simulink model "MAIN_UAVSIM_Simulink"  (R2022a)
settings: Solver=FixedStepAuto  StartTime=0.0  StopTime=inf  RelTol=1e-3  EnableMultiTasking=on
undefined symbols (not defined in the file or in its folder): altREF, latREF, lonREF
libraries: slrealtimeutilitieslib x3, dspnetwork x2, slrealtimeiplib x1, aerolibanimutils x1, deeplib x1
settings Model: Creator=WiSE EFS  LastModifiedBy=Adi Kelvianto
settings SolverCC: AlgebraicLoopSolver=TrustRegion
settings DataIOCC: SaveFormat=Array  SignalLoggingSaveFormat=ModelDataLogs  SaveOutput=off  SaveTime=off  ReturnWorkspaceOutputs=off
settings OptimizationCC: ExpressionDepthLimit=2147483647  LifeSpan=inf
settings DebuggingCC: UnderspecifiedInitializationDetection=Classic  MergeDetectMultiDrivingBlocksExec=none  SolverPrmCheckMsg=warning  InheritedTsInSrcMsg=none  MultiTaskCondExecSysMsg=none  MultiTaskRateTransMsg=warning  SigSpecEnsureSampleTimeMsg=none  FcnCallInpInsideContextMsg=warning  UnconnectedInputMsg=warning  UnconnectedOutputMsg=warning  UnconnectedLineMsg=warning  StateNameClashWarn=warning  SFUnexpectedBacktrackingDiag=warning  SFNoUnconditionalDefaultTransitionDiag=warning  SFExecutionAtInitializationDiag=none  SFMachineParentedDataDiag=warning  ArithmeticOperatorsInVariantConditions=warning
settings HardwareCC: ProdBitPerPointer=32  ProdBitPerSizeT=32  ProdBitPerPtrDiffT=32  ProdLargestAtomicFloat=None  ProdIntDivRoundTo=Undefined  ProdEndianess=Unspecified  ProdWordSize=32  ProdHWDeviceType=32-bit Generic
settings ModelReferenceCC: PropagateSignalLabelsOutOfModel=off
settings SFSimCC: SimUseLocalCustomCode=off  SimParseCustomCode=off  CustomCodeUndefinedFunction=UseInterfaceOnly  SimTargetLang=C++
settings RTWCC: RTWUseLocalCustomCode=off  TargetLang=C++  DLArmComputeVersion=19.05
settings CodeAppCC: StateflowObjectComments=on
settings GRTTargetCC: TargetLangStandard=C89/C90 (ANSI)  CombineOutputUpdateFcns=off  GRTInterface=on
settings ConfigComp: CovMetricSettings=dw  CovSaveCumulativeToWorkspaceVar=on  CovSaveSingleToWorkspaceVar=on  CovExternalEMLEnable=off  CovSFcnEnable=off

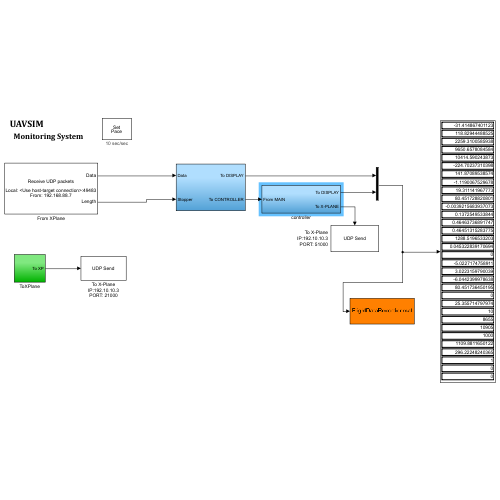
[thumbnail: Simulink's stored preview of the top-level diagram]
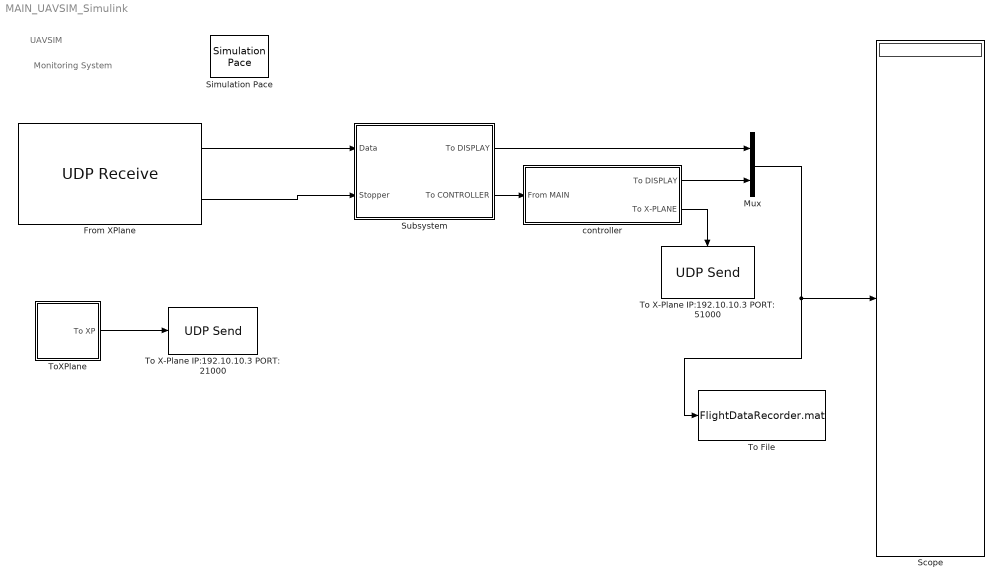
== system MAIN_UAVSIM_Simulink ==
  note: UAVSIM
  note: Monitoring System
  From XPlane : slrealtimeiplib/UDP Receive  useHostTargetConn=on  ipAddress=10.10.10.15  localPort=49483  rcvWidth=80  rcvFmAny=off  fmAddress=192.168.88.7  sampleTime=-1  enableMessage=off  maxPackets=1
      settings: SourceProductBaseCode=XP
  Mux : Mux  Inputs=2
  Scope : Display
  Simulation Pace : aerolibanimutils/Simulation Pace  SimulationPace=10  SleepMode=MATLAB Thread  OutputPaceError=off  SampleTime=-1
      settings: AttributesFormatString=%<SimulationPace> sec/sec
  Subsystem : Subsystem
  To File : ToFile  Filename=FlightDataRecorder.mat  MatrixName=FlightData  SampleTime=0.02
      settings: Decimation=50
  To X-Plane IP:192.10.10.3 PORT: 21000 : dspnetwork/UDP Send  remoteURL='192.168.88.7'  remotePort=49001  localURL='0.0.0.0'  localPortSource=Automatically determine  localPort=-1  sendBufferSize=8192  sampletime=-1  blockPlatform=[]  separateLengthPort=0
  To X-Plane IP:192.10.10.3 PORT: 51000 : dspnetwork/UDP Send  remoteURL='192.168.88.7'  remotePort=49000  localURL='0.0.0.0'  localPortSource=Automatically determine  localPort=-1  sendBufferSize=8192  sampletime=-1  blockPlatform=[]  separateLengthPort=0
  ToXPlane : Subsystem
  controller : Subsystem
  wires:
  From XPlane/1 -> Subsystem/1(Data)
  From XPlane/2 -> Subsystem/2(Stopper)
  ToXPlane/1(To XP) -> To X-Plane IP:192.10.10.3 PORT: 21000/1
  Subsystem/2(To CONTROLLER) -> controller/1(From MAIN)
  controller/2(To X-PLANE) -> To X-Plane IP:192.10.10.3 PORT: 51000/1
  Subsystem/1(To DISPLAY) -> Mux/1
  controller/1(To DISPLAY) -> Mux/2
  Mux/1 -> To File/1, Scope/1

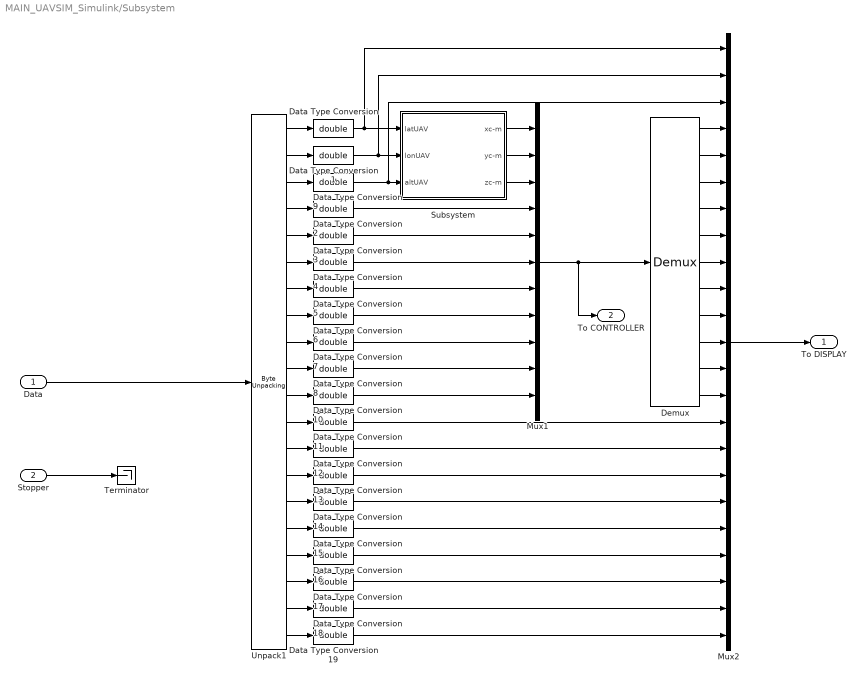
== system MAIN_UAVSIM_Simulink/Subsystem ==
  Data : Inport
  Stopper : Inport  Port=2
  Data Type Conversion{,1..19} (20 alike) : DataTypeConversion  OutDataTypeStr=double  SaturateOnIntegerOverflow=off  RndMeth=Floor
  Demux : Demux  Outputs=11
      settings: DisplayOption=none
  Mux1 : Mux  Inputs=11
  Mux2 : Mux  Inputs=23
  Subsystem : Subsystem
  Terminator : Terminator
  Unpack1 : slrealtimeutilitieslib/Byte Unpacking  MaskUnpackedDataTypes=dataType  MaskUnpackedDataSizes=dataChannel  MaskAlignment=4
      settings: SourceProductBaseCode=XP
  To DISPLAY : Outport
  To CONTROLLER : Outport  Port=2
  wires:
  Data/1 -> Unpack1/1
  Stopper/1 -> Terminator/1
  Unpack1/1 -> Data Type Conversion/1
  Unpack1/2 -> Data Type Conversion1/1
  Unpack1/3 -> Data Type Conversion9/1
  Unpack1/4 -> Data Type Conversion2/1
  Unpack1/5 -> Data Type Conversion3/1
  Unpack1/6 -> Data Type Conversion4/1
  Data Type Conversion1/1 -> Mux2/2, Subsystem/2(lonUAV)
  Data Type Conversion9/1 -> Mux2/3, Subsystem/3(altUAV)
  Subsystem/1(xc-m) -> Mux1/1
  Subsystem/2(yc-m) -> Mux1/2
  Subsystem/3(zc-m) -> Mux1/3
  Data Type Conversion2/1 -> Mux1/4
  Data Type Conversion3/1 -> Mux1/5
  Data Type Conversion4/1 -> Mux1/6
  Unpack1/7 -> Data Type Conversion5/1
  Unpack1/8 -> Data Type Conversion6/1
  Data Type Conversion6/1 -> Mux1/8
  Unpack1/9 -> Data Type Conversion7/1
  Data Type Conversion7/1 -> Mux1/9
  Unpack1/10 -> Data Type Conversion8/1
  Data Type Conversion8/1 -> Mux1/10
  Unpack1/11 -> Data Type Conversion10/1
  Data Type Conversion10/1 -> Mux1/11
  Unpack1/12 -> Data Type Conversion11/1
  Unpack1/13 -> Data Type Conversion12/1
  Unpack1/14 -> Data Type Conversion13/1
  Unpack1/15 -> Data Type Conversion14/1
  Unpack1/16 -> Data Type Conversion15/1
  Unpack1/17 -> Data Type Conversion16/1
  Unpack1/18 -> Data Type Conversion17/1
  Unpack1/19 -> Data Type Conversion18/1
  Unpack1/20 -> Data Type Conversion19/1
  Mux2/1 -> To DISPLAY/1
  Data Type Conversion5/1 -> Mux1/7
  Data Type Conversion/1 -> Mux2/1, Subsystem/1(latUAV)
  Data Type Conversion19/1 -> Mux2/23
  Data Type Conversion18/1 -> Mux2/22
  Data Type Conversion17/1 -> Mux2/21
  Data Type Conversion16/1 -> Mux2/20
  Data Type Conversion15/1 -> Mux2/19
  Data Type Conversion14/1 -> Mux2/18
  Data Type Conversion13/1 -> Mux2/17
  Data Type Conversion12/1 -> Mux2/16
  Data Type Conversion11/1 -> Mux2/15
  Mux1/1 -> To CONTROLLER/1, Demux/1
  Demux/11 -> Mux2/14
  Demux/10 -> Mux2/13
  Demux/9 -> Mux2/12
  Demux/8 -> Mux2/11
  Demux/7 -> Mux2/10
  Demux/6 -> Mux2/9
  Demux/5 -> Mux2/8
  Demux/4 -> Mux2/7
  Demux/3 -> Mux2/6
  Demux/2 -> Mux2/5
  Demux/1 -> Mux2/4

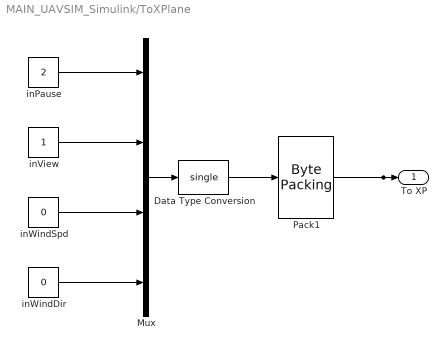
== system MAIN_UAVSIM_Simulink/ToXPlane ==
  Data Type Conversion : DataTypeConversion  OutDataTypeStr=single  SaturateOnIntegerOverflow=off  RndMeth=Floor
  Mux : Mux
  Pack1 : slrealtimeutilitieslib/Byte Packing  MaskPackedDataType=uint8  MaskUnpackedDataTypes={'single'}  MaskAlignment=4
  inPause : Constant  Value=2  SampleTime=0
  inView : Constant  SampleTime=0
  inWindDir : Constant  Value=0  SampleTime=0
  inWindSpd : Constant  Value=0  SampleTime=0
  To XP : Outport
  wires:
  Mux/1 -> Data Type Conversion/1
  Pack1/1 -> To XP/1
  inPause/1 -> Mux/1
  inView/1 -> Mux/2
  inWindSpd/1 -> Mux/3
  inWindDir/1 -> Mux/4
  Data Type Conversion/1 -> Pack1/1

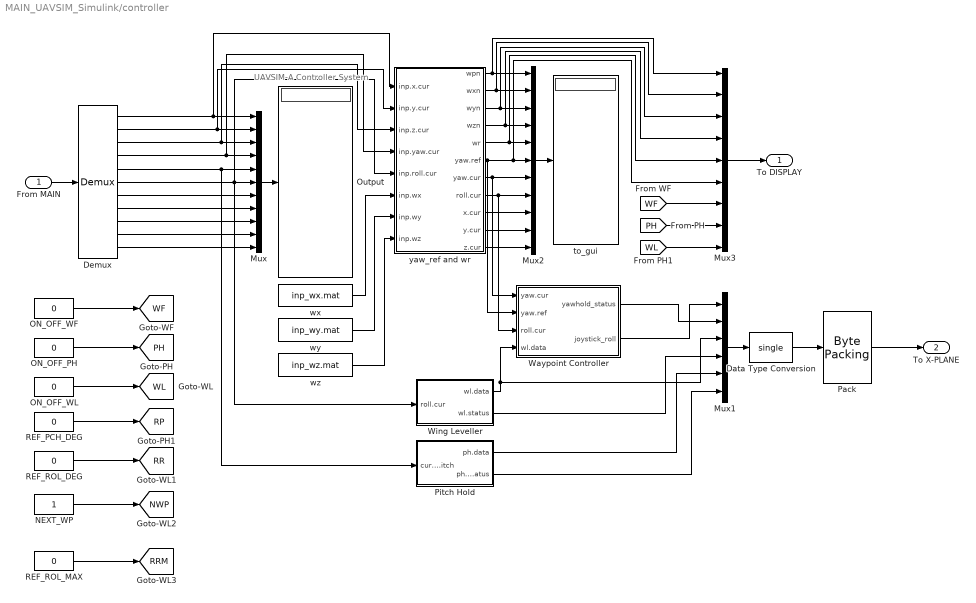
== system MAIN_UAVSIM_Simulink/controller ==
  note: UAVSIM-A
      | Controller System
  From MAIN : Inport
  Data Type Conversion : DataTypeConversion  OutDataTypeStr=single  SaturateOnIntegerOverflow=off  RndMeth=Floor
  Demux : Demux  Outputs=11
      settings: DisplayOption=none
  Mux : Mux  Inputs=11
  Mux1 : Mux  Inputs=6
  Mux2 : Mux  Inputs=11
  Mux3 : Mux  Inputs=9
  NEXT_WP : Constant  SampleTime=0
  ON_OFF_PH : Constant  Value=0  SampleTime=0
  ON_OFF_WF : Constant  Value=0  SampleTime=0
  ON_OFF_WL : Constant  Value=0  SampleTime=0
  Output : Display
  Pack : slrealtimeutilitieslib/Byte Packing  MaskPackedDataType=uint8  MaskUnpackedDataTypes={'single'}  MaskAlignment=4
  Pitch Hold : Subsystem
  REF_PCH_DEG : Constant  Value=0  SampleTime=0
  REF_ROL_DEG : Constant  Value=0  SampleTime=0
  REF_ROL_MAX : Constant  Value=0  SampleTime=0
  Waypoint Controller : Subsystem
  Wing Leveller : Subsystem
  to_gui : Display
  wx : FromFile  FileName=inp_wx.mat  SampleTime=0  ExtrapolationBeforeFirstDataPoint=Hold first value  ExtrapolationAfterLastDataPoint=Hold last value
  wy : FromFile  FileName=inp_wy.mat  SampleTime=0  ExtrapolationBeforeFirstDataPoint=Hold first value  ExtrapolationAfterLastDataPoint=Hold last value
  wz : FromFile  FileName=inp_wz.mat  SampleTime=0  ExtrapolationBeforeFirstDataPoint=Hold first value  ExtrapolationAfterLastDataPoint=Hold last value
  yaw_ref and wr : Subsystem
  To DISPLAY : Outport
  To X-PLANE : Outport  Port=2
  tag scope: NWP=global, PH=global, RP=global, RR=global, RRM=global, WF=global, WL=global
  wires:
  yaw_ref and wr/10(y.cur) -> Mux2/10
  yaw_ref and wr/9(x.cur) -> Mux2/9
  Waypoint Controller/1(yawhold_status) -> Mux1/2
  yaw_ref and wr/7(yaw.cur) -> Waypoint Controller/1(yaw.cur), Mux2/7
  Wing Leveller/2(wl.status) -> Mux1/4
  Wing Leveller/1(wl.data) -> Waypoint Controller/4(wl.data), Mux1/3
  ON_OFF_WL/1 -> [WL]
  ON_OFF_WF/1 -> [WF]
  yaw_ref and wr/5(wr) -> Mux2/5, Mux3/5
  yaw_ref and wr/2(wxn) -> Mux2/2, Mux3/2
  Mux/1 -> Output/1
  Demux/11 -> Mux/11
  Mux1/1 -> Data Type Conversion/1
  REF_PCH_DEG/1 -> [RP]
  Demux/1 -> Mux/1, yaw_ref and wr/1(inp.x.cur)
  yaw_ref and wr/11(z.cur) -> Mux2/11
  wz/1 -> yaw_ref and wr/8(inp.wz)
  NEXT_WP/1 -> [NWP]
  Demux/7 -> Mux/7
  yaw_ref and wr/8(roll.cur) -> Waypoint Controller/3(roll.cur), Mux2/8
  yaw_ref and wr/4(wzn) -> Mux2/4, Mux3/4
  Demux/2 -> Mux/2, yaw_ref and wr/2(inp.y.cur)
  [WL] -> Mux3/9
  Pitch Hold/2(ph.status) -> Mux1/6
  Mux2/1 -> to_gui/1
  Demux/5 -> Mux/5, Pitch Hold/1(cur.pitch)
  Demux/8 -> Mux/8
  REF_ROL_DEG/1 -> [RR]
  wx/1 -> yaw_ref and wr/6(inp.wx)
  Demux/4 -> Mux/4, yaw_ref and wr/4(inp.yaw.cur)
  Waypoint Controller/2(joystick_roll) -> Mux1/1
  yaw_ref and wr/6(yaw.ref) -> Waypoint Controller/2(yaw.ref), Mux2/6, Mux3/6
  Demux/3 -> Mux/3, yaw_ref and wr/3(inp.z.cur)
  Pitch Hold/1(ph.data) -> Mux1/5
  Demux/6 -> Mux/6, Wing Leveller/1(roll.cur), yaw_ref and wr/5(inp.roll.cur)
  wy/1 -> yaw_ref and wr/7(inp.wy)
  Data Type Conversion/1 -> Pack/1
  ON_OFF_PH/1 -> [PH]
  yaw_ref and wr/1(wpn) -> Mux2/1, Mux3/1
  Demux/9 -> Mux/9
  Demux/10 -> Mux/10
  [WF] -> Mux3/7
  [PH] -> Mux3/8
  yaw_ref and wr/3(wyn) -> Mux2/3, Mux3/3
  From MAIN/1 -> Demux/1
  Mux3/1 -> To DISPLAY/1
  Pack/1 -> To X-PLANE/1
  REF_ROL_MAX/1 -> [RRM]

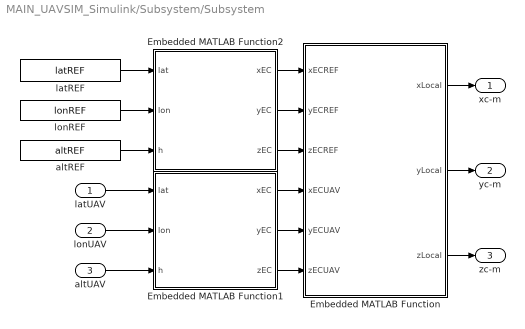
== system MAIN_UAVSIM_Simulink/Subsystem/Subsystem ==
  latUAV : Inport
  lonUAV : Inport  Port=2
  altUAV : Inport  Port=3
  Embedded MATLAB Function : MATLAB Function  TreatAsAtomicUnit=on
  Embedded MATLAB Function1 : MATLAB Function  TreatAsAtomicUnit=on
  Embedded MATLAB Function2 : MATLAB Function  TreatAsAtomicUnit=on
  altREF : Constant  Value=altREF  SampleTime=0.02
  latREF : Constant  Value=latREF  SampleTime=0.02
  lonREF : Constant  Value=lonREF  SampleTime=0.02
  xc-m : Outport
  yc-m : Outport  Port=2
  zc-m : Outport  Port=3
  wires:
  Embedded MATLAB Function/1(xLocal) -> xc-m/1
  Embedded MATLAB Function/3(zLocal) -> zc-m/1
  Embedded MATLAB Function/2(yLocal) -> yc-m/1
  latREF/1 -> Embedded MATLAB Function2/1(lat)
  lonREF/1 -> Embedded MATLAB Function2/2(lon)
  altREF/1 -> Embedded MATLAB Function2/3(h)
  Embedded MATLAB Function2/1(xEC) -> Embedded MATLAB Function/1(xECREF)
  Embedded MATLAB Function2/2(yEC) -> Embedded MATLAB Function/2(yECREF)
  Embedded MATLAB Function2/3(zEC) -> Embedded MATLAB Function/3(zECREF)
  Embedded MATLAB Function1/1(xEC) -> Embedded MATLAB Function/4(xECUAV)
  Embedded MATLAB Function1/2(yEC) -> Embedded MATLAB Function/5(yECUAV)
  Embedded MATLAB Function1/3(zEC) -> Embedded MATLAB Function/6(zECUAV)
  latUAV/1 -> Embedded MATLAB Function1/1(lat)
  lonUAV/1 -> Embedded MATLAB Function1/2(lon)
  altUAV/1 -> Embedded MATLAB Function1/3(h)

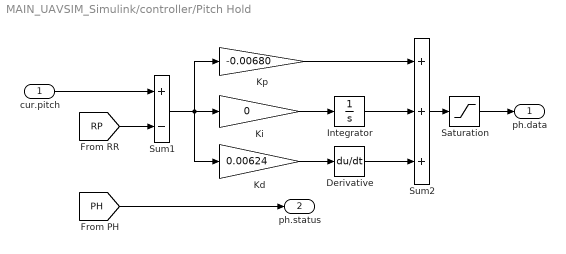
== system MAIN_UAVSIM_Simulink/controller/Pitch Hold ==
  cur.pitch : Inport
  Derivative : Derivative
  Integrator : Integrator
  Kd : Gain  Gain=0.00624
  Ki : Gain  Gain=0
  Kp : Gain  Gain=-0.00680
  Saturation : Saturate  UpperLimit=1  LowerLimit=-1
  Sum1 : Sum  Inputs=+-
  Sum2 : Sum  Inputs=+++
  ph.data : Outport
  ph.status : Outport  Port=2
  wires:
  Integrator/1 -> Sum2/2
  Ki/1 -> Integrator/1
  Kp/1 -> Sum2/1
  Sum2/1 -> Saturation/1
  Kd/1 -> Derivative/1
  Derivative/1 -> Sum2/3
  [PH] -> ph.status/1
  Sum1/1 -> Ki/1, Kp/1, Kd/1
  cur.pitch/1 -> Sum1/1
  Saturation/1 -> ph.data/1
  [RP] -> Sum1/2

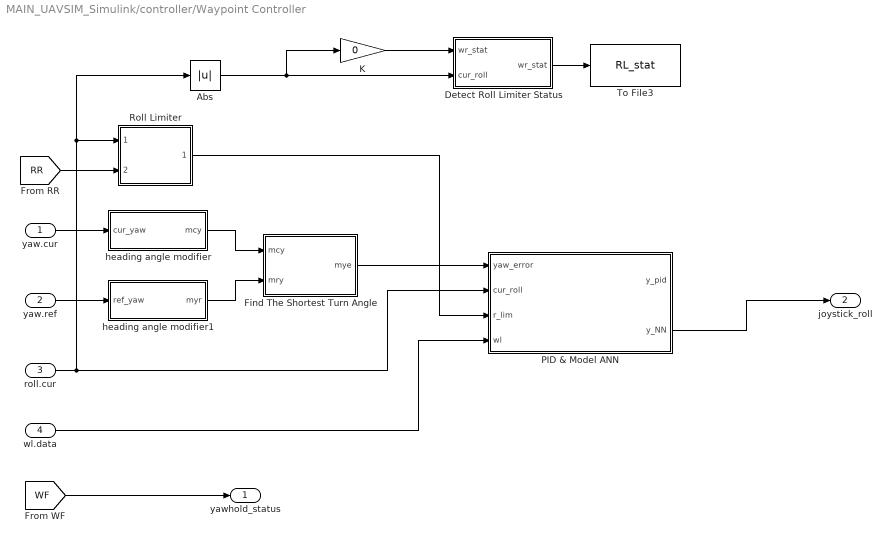
== system MAIN_UAVSIM_Simulink/controller/Waypoint Controller ==
  yaw.cur : Inport
  yaw.ref : Inport  Port=2
  roll.cur : Inport  Port=3
  wl.data : Inport  Port=4
  Abs : Abs  SaturateOnIntegerOverflow=off
  Detect Roll Limiter Status : MATLAB Function  TreatAsAtomicUnit=on
  Find The Shortest Turn Angle : MATLAB Function  TreatAsAtomicUnit=on
  K : Gain  Gain=0
  PID & Model ANN : Subsystem
  Roll Limiter : Subsystem
  To File3 : ToFile  Filename=RL_stat  MatrixName=RL_stat  SampleTime=0.02
      settings: Decimation=50
  heading angle modifier : MATLAB Function  TreatAsAtomicUnit=on
  heading angle modifier1 : MATLAB Function  TreatAsAtomicUnit=on
  yawhold_status : Outport
  joystick_roll : Outport  Port=2
  wires:
  [WF] -> yawhold_status/1
  [RR] -> Roll Limiter/2(roll.ref.max)
  yaw.cur/1 -> heading angle modifier/1(cur_yaw)
  yaw.ref/1 -> heading angle modifier1/1(ref_yaw)
  K/1 -> Detect Roll Limiter Status/1("wr_stat ")
  roll.cur/1 -> Abs/1, Roll Limiter/1(roll.cur), PID & Model ANN/2(cur_roll)
  Abs/1 -> K/1, Detect Roll Limiter Status/2(cur_roll)
  Detect Roll Limiter Status/1(wr_stat) -> To File3/1
  wl.data/1 -> PID & Model ANN/4(wl)
  Roll Limiter/1(roll.lim) -> PID & Model ANN/3(r_lim)
  heading angle modifier/1(mcy) -> Find The Shortest Turn Angle/1(mcy)
  heading angle modifier1/1(myr) -> Find The Shortest Turn Angle/2(mry)
  Find The Shortest Turn Angle/1(mye) -> PID & Model ANN/1(yaw_error)
  PID & Model ANN/2(y_NN) -> joystick_roll/1

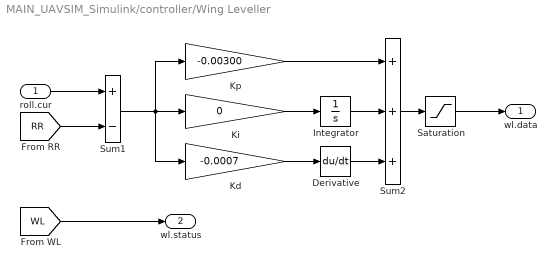
== system MAIN_UAVSIM_Simulink/controller/Wing Leveller ==
  roll.cur : Inport
  Derivative : Derivative
  Integrator : Integrator
  Kd : Gain  Gain=-0.0007
  Ki : Gain  Gain=0
  Kp : Gain  Gain=-0.00300
  Saturation : Saturate  UpperLimit=1  LowerLimit=-1
  Sum1 : Sum  Inputs=+-
  Sum2 : Sum  Inputs=+++
  wl.data : Outport
  wl.status : Outport  Port=2
  wires:
  Integrator/1 -> Sum2/2
  Ki/1 -> Integrator/1
  Kp/1 -> Sum2/1
  Sum2/1 -> Saturation/1
  Kd/1 -> Derivative/1
  Derivative/1 -> Sum2/3
  Sum1/1 -> Ki/1, Kp/1, Kd/1
  [RR] -> Sum1/2
  roll.cur/1 -> Sum1/1
  Saturation/1 -> wl.data/1
  [WL] -> wl.status/1

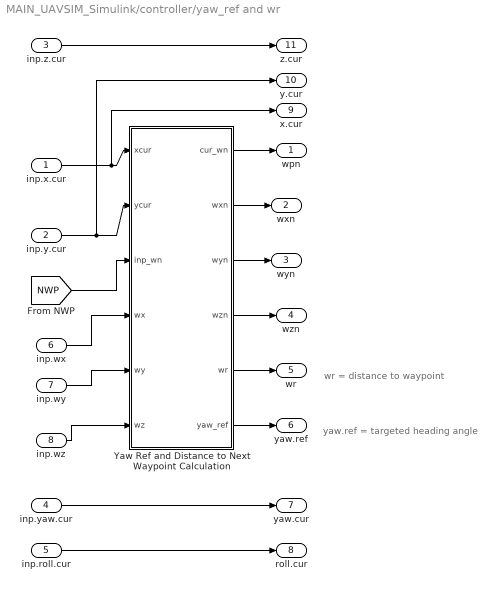
== system MAIN_UAVSIM_Simulink/controller/yaw_ref and wr ==
  note: yaw.ref = targeted heading angle
  note: wr = distance to waypoint
  inp.x.cur : Inport
  inp.y.cur : Inport  Port=2
  inp.z.cur : Inport  Port=3
  inp.yaw.cur : Inport  Port=4
  inp.roll.cur : Inport  Port=5
  inp.wx : Inport  Port=6
  inp.wy : Inport  Port=7
  inp.wz : Inport  Port=8
  Yaw Ref and Distance to Next Waypoint Calculation : MATLAB Function  TreatAsAtomicUnit=on
  wpn : Outport
  wxn : Outport  Port=2
  wyn : Outport  Port=3
  wzn : Outport  Port=4
  wr : Outport  Port=5
  yaw.ref : Outport  Port=6
  yaw.cur : Outport  Port=7
  roll.cur : Outport  Port=8
  x.cur : Outport  Port=9
  y.cur : Outport  Port=10
  z.cur : Outport  Port=11
  wires:
  inp.y.cur/1 -> Yaw Ref and Distance to Next Waypoint Calculation/2(ycur), y.cur/1
  inp.x.cur/1 -> Yaw Ref and Distance to Next Waypoint Calculation/1(xcur), x.cur/1
  [NWP] -> Yaw Ref and Distance to Next Waypoint Calculation/3(inp_wn)
  inp.yaw.cur/1 -> yaw.cur/1
  Yaw Ref and Distance to Next Waypoint Calculation/6(yaw_ref) -> yaw.ref/1
  inp.roll.cur/1 -> roll.cur/1
  Yaw Ref and Distance to Next Waypoint Calculation/1(cur_wn) -> wpn/1
  Yaw Ref and Distance to Next Waypoint Calculation/2(wxn) -> wxn/1
  Yaw Ref and Distance to Next Waypoint Calculation/3(wyn) -> wyn/1
  Yaw Ref and Distance to Next Waypoint Calculation/4(wzn) -> wzn/1
  Yaw Ref and Distance to Next Waypoint Calculation/5(wr) -> wr/1
  inp.z.cur/1 -> z.cur/1
  inp.wx/1 -> Yaw Ref and Distance to Next Waypoint Calculation/4(wx)
  inp.wy/1 -> Yaw Ref and Distance to Next Waypoint Calculation/5(wy)
  inp.wz/1 -> Yaw Ref and Distance to Next Waypoint Calculation/6(wz)

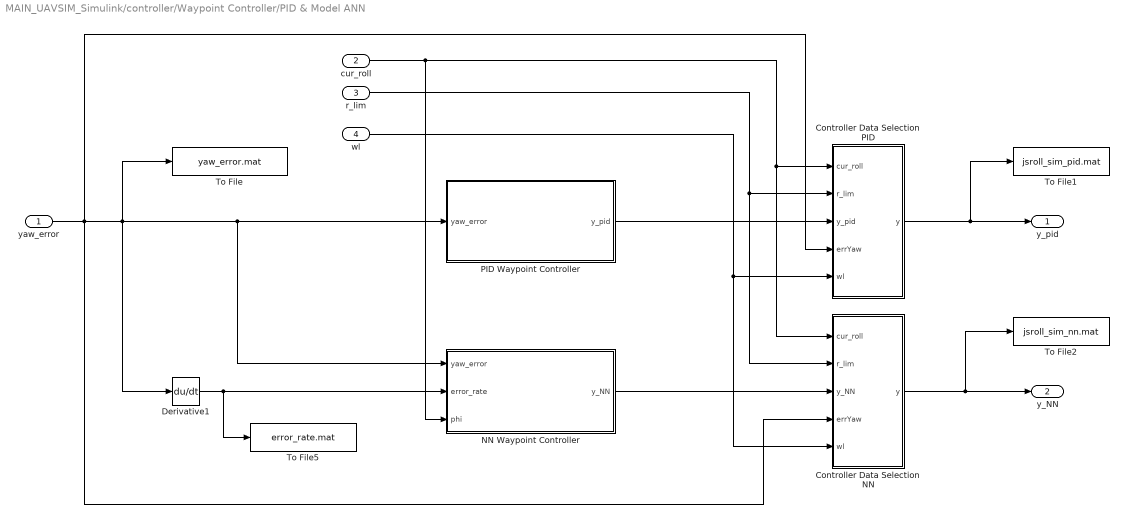
== system MAIN_UAVSIM_Simulink/controller/Waypoint Controller/PID & Model ANN ==
  yaw_error : Inport
  cur_roll : Inport  Port=2
  r_lim : Inport  Port=3
  wl : Inport  Port=4
  Controller Data Selection NN : MATLAB Function  TreatAsAtomicUnit=on
  Controller Data Selection PID : MATLAB Function  TreatAsAtomicUnit=on
  Derivative1 : Derivative
  NN Waypoint Controller : Subsystem
  PID Waypoint Controller : Subsystem
  To File : ToFile  Filename=yaw_error.mat  MatrixName=yaw_error  SampleTime=0.02
      settings: Decimation=50
  To File1 : ToFile  Filename=jsroll_sim_pid.mat  MatrixName=jsroll_sim_pid  SampleTime=0.02
      settings: Decimation=50
  To File2 : ToFile  Filename=jsroll_sim_nn.mat  MatrixName=jsroll_sim_nn  SampleTime=0.02
      settings: Decimation=50
  To File5 : ToFile  Filename=error_rate.mat  MatrixName=error_rate  SampleTime=0.02
      settings: Decimation=50
  y_pid : Outport
  y_NN : Outport  Port=2
  wires:
  PID Waypoint Controller/1(y_pid) -> Controller Data Selection PID/3(y_pid)
  cur_roll/1 -> Controller Data Selection NN/1(cur_roll), Controller Data Selection PID/1(cur_roll), NN Waypoint Controller/3(phi)
  r_lim/1 -> Controller Data Selection NN/2(r_lim), Controller Data Selection PID/2(r_lim)
  wl/1 -> Controller Data Selection NN/5(wl), Controller Data Selection PID/5(wl)
  NN Waypoint Controller/1(y_NN) -> Controller Data Selection NN/3(y_NN)
  Controller Data Selection PID/1(y) -> To File1/1, y_pid/1
  Controller Data Selection NN/1(y) -> To File2/1, y_NN/1
  yaw_error/1 -> Controller Data Selection NN/4(errYaw), Controller Data Selection PID/4(errYaw), To File/1, Derivative1/1, NN Waypoint Controller/1(yaw_error), PID Waypoint Controller/1(yaw_error)
  Derivative1/1 -> To File5/1, NN Waypoint Controller/2(error_rate)

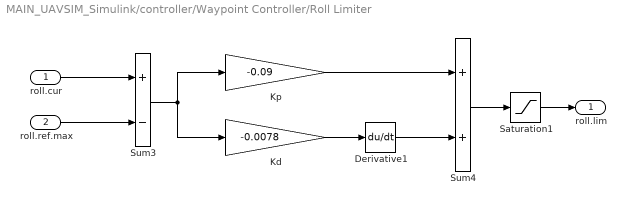
== system MAIN_UAVSIM_Simulink/controller/Waypoint Controller/Roll Limiter ==
  roll.cur : Inport
  roll.ref.max : Inport  Port=2
  Derivative1 : Derivative
  Kd : Gain  Gain=-0.0078
  Kp : Gain  Gain=-0.09
  Saturation1 : Saturate  UpperLimit=1  LowerLimit=-1
  Sum3 : Sum  Inputs=+-
  Sum4 : Sum
  roll.lim : Outport
  wires:
  Sum3/1 -> Kp/1, Kd/1
  Sum4/1 -> Saturation1/1
  Saturation1/1 -> roll.lim/1
  Derivative1/1 -> Sum4/2
  roll.ref.max/1 -> Sum3/2
  Kp/1 -> Sum4/1
  Kd/1 -> Derivative1/1
  roll.cur/1 -> Sum3/1

== system MAIN_UAVSIM_Simulink/controller/Waypoint Controller/PID & Model ANN/NN Waypoint Controller ==
  yaw_error : Inport
  error_rate : Inport  Port=2
  phi : Inport  Port=3
  Predict : deeplib/Predict  Network=Network from MAT-file  NetworkFunction=squeezenet  NetworkFilePath=D:\uavms\model_7aug_set4.mat  MiniBatchSize=1  InputDataFormats={ '', '' }  Predictions=on  Activations={}  ForceInterpretedSim=off  EnableDLNetwork=on
      settings: SourceProductBaseCode=NN
  Prepare Features : MATLAB Function  TreatAsAtomicUnit=on
  Saturation1 : Saturate  UpperLimit=1  LowerLimit=-1
  y_NN : Outport
  wires:
  error_rate/1 -> Prepare Features/1(error_rate)
  yaw_error/1 -> Prepare Features/2(yaw_error)
  phi/1 -> Prepare Features/3(phi)
  Prepare Features/1(features) -> Predict/1
  Saturation1/1 -> y_NN/1
  Predict/1 -> Saturation1/1

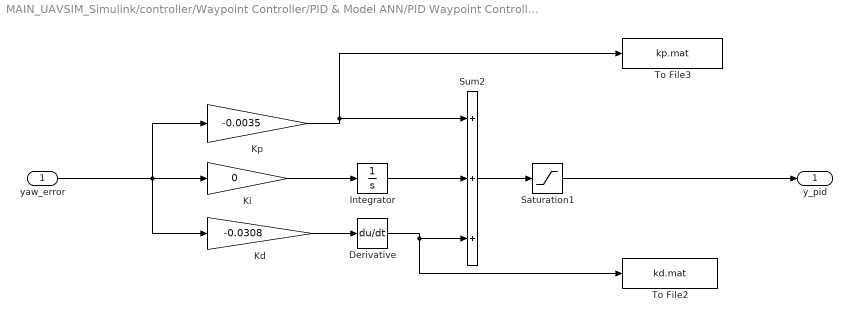
== system MAIN_UAVSIM_Simulink/controller/Waypoint Controller/PID & Model ANN/PID Waypoint Controller ==
  yaw_error : Inport
  Derivative : Derivative
  Integrator : Integrator
  Kd : Gain  Gain=-0.0308
  Ki : Gain  Gain=0
  Kp : Gain  Gain=-0.0035
  Saturation1 : Saturate  UpperLimit=1  LowerLimit=-1
  Sum2 : Sum  Inputs=+++
  To File2 : ToFile  Filename=kd.mat  MatrixName=kd  SampleTime=0.02
      settings: Decimation=50
  To File3 : ToFile  Filename=kp.mat  MatrixName=kp  SampleTime=0.02
      settings: Decimation=50
  y_pid : Outport
  wires:
  Sum2/1 -> Saturation1/1
  Derivative/1 -> Sum2/3, To File2/1
  Kp/1 -> To File3/1, Sum2/1
  Saturation1/1 -> y_pid/1
  Kd/1 -> Derivative/1
  yaw_error/1 -> Kd/1, Ki/1, Kp/1
  Ki/1 -> Integrator/1
  Integrator/1 -> Sum2/2

== matlab function MAIN_UAVSIM_Simulink/controller/yaw_ref and wr/Yaw Ref and Distance to Next Waypoint Calculation ==
  data: cur_wn output; wxn output; wyn output; wzn output; wr output; xcur input; yaw_ref output; ycur input; inp_wn input; wx input; wy input; wz input
function [cur_wn,wxn,wyn,wzn,wr,yaw_ref]  = fcn(xcur,ycur,inp_wn,wx,wy,wz)
%#eml

% Rectangular Waypoint
% wx = [3000;3000;8000;8000;3000;3000]; % The last data is for terminating only
% wy = [2000;8000;8000;2000;2000;2000]; % The last data is for terminating only
% wz = [500;600;500;500;500;700];

% Rectangular + X Waypoint
% wx = [3000;8000;3000;8000;3000;3000]; % The last data is for terminating only
% wy = [2000;2000;8000;8000;2000;2000]; % The last data is for terminating only
% wz = [500;600;500;500;500;700];

% Next waypoint coordinate
wxn = wx(inp_wn);
wyn = wy(inp_wn);
wzn = wz(inp_wn);

dx  = wx(inp_wn)-xcur;
dy  = wy(inp_wn)-ycur;

% Next waypoint heading angle and distance
yaw = 180*(atan2(dy,dx))/pi;
wr  = sqrt(dx^2 + dy^2);
    
if (dx < 0 && dy > 0)
    yaw_ref = 360 + (90-yaw);
else
    yaw_ref = 90-yaw;
end
   
cur_wn = inp_wn;

== matlab function MAIN_UAVSIM_Simulink/controller/Waypoint Controller/PID & Model ANN/NN Waypoint Controller/Prepare Features ==
  data: error_rate input; yaw_error input; features output; phi input
function features = fcn(error_rate, yaw_error, phi)
%#eml

features_raw = [error_rate, yaw_error,phi];
% Min Max value from train dataset for each features with sequnce of
% [error_rate, yaw_error, phi]

% set 1
%min_train = [-2.101, -17.924, -8.977];
%max_train = [1.543, 17.016, 9.541];

% set 2
%min_train = [-2.331, -93.562, -8.977];
%max_train = [5.371, 17.016, 32.265];

% set 3
%min_train = [-6.707, -17.924, -32.134];
%max_train = [4.487, 71.031, 9.541];

% set 4
min_train = [-6.707, -93.562, -32.134] ;
max_train = [5.559, 71.031, 34.303] ;

normalized = zeros(1,length(features_raw));

for i = 1:length(features_raw)
    normalized(i) = (features_raw(i)-min_train(i))/(max_train(i)-min_train(i));
end

features = normalized;
end

== matlab function MAIN_UAVSIM_Simulink/controller/Waypoint Controller/PID & Model ANN/Controller Data Selection NN ==
  data: cur_roll input; r_lim input; y output; y_NN input; errYaw input; wl input
function y = fcn(cur_roll,r_lim,y_NN,errYaw,wl)
%#eml
%diff

if abs(cur_roll)>=30
    y = r_lim;
else
    y = double(y_NN);
end
end

== matlab function MAIN_UAVSIM_Simulink/Subsystem/Subsystem/Embedded MATLAB Function1 ==
  data: lat input; lon input; xEC output; h input; yEC output; zEC output
function [xEC,yEC,zEC] = WGS2ECEF(lat,lon,h)

% Convert lat, long, height in WGS84 to ECEF X,Y,Z
% lat and long given in decimal degrees.
% altitude should be given in meters
a  = 6378137.0;       % earth semimajor axis in meters
f  = 1/298.257223563; % reciprocal flattening
e2 = 2*f -f^2;        % eccentricity squared
 
chi = sqrt(1-e2*(sind(lat)).^2);
xEC = (a./chi + h).*cosd(lat).*cosd(lon);
yEC = (a./chi + h).*cosd(lat).*sind(lon);
zEC = (a*(1-e2)./chi + h).*sind(lat);

== matlab function MAIN_UAVSIM_Simulink/Subsystem/Subsystem/Embedded MATLAB Function ==
  data: xLocal output; xECREF input; yECREF input; zECREF input; yLocal output; zLocal output; xECUAV input; yECUAV input; zECUAV input
function [xLocal,yLocal,zLocal] = ECEF2LOC(xECREF,yECREF,zECREF,xECUAV,yECUAV,zECUAV)

% convert ECEF coordinates to local east, north, up

phiP = atan2(zECREF,sqrt(xECREF^2 + yECREF^2));
lambda = atan2(yECREF,xECREF);
 
xLocal = -sin(lambda).*(xECUAV-xECREF) + cos(lambda).*(yECUAV-yECREF);
yLocal = -sin(phiP).*cos(lambda).*(xECUAV-xECREF) - sin(phiP).*sin(lambda)...
          .*(yECUAV-yECREF) + cos(phiP).*(zECUAV-zECREF);
zLocal = cos(phiP).*cos(lambda).*(xECUAV-xECREF) + cos(phiP).*sin(lambda)...
          .*(yECUAV-yECREF) + sin(phiP).*(zECUAV-zECREF);

== matlab function MAIN_UAVSIM_Simulink/Subsystem/Subsystem/Embedded MATLAB Function2 ==
  data: lat input; lon input; xEC output; h input; yEC output; zEC output
function [xEC,yEC,zEC] = WGS2ECEF(lat,lon,h)

% Convert lat, long, height in WGS84 to ECEF X,Y,Z
% lat and long given in decimal degrees.
% altitude should be given in meters
a  = 6378137.0;       % earth semimajor axis in meters
f  = 1/298.257223563; % reciprocal flattening
e2 = 2*f -f^2;        % eccentricity squared
 
chi = sqrt(1-e2*(sind(lat)).^2);
xEC = (a./chi + h).*cosd(lat).*cosd(lon);
yEC = (a./chi + h).*cosd(lat).*sind(lon);
zEC = (a*(1-e2)./chi + h).*sind(lat);

== matlab function MAIN_UAVSIM_Simulink/controller/Waypoint Controller/Find The Shortest Turn Angle ==
  data: mcy input; mye output; mry input
function mye = fcn(mcy,mry)
%#eml
% mye = modified yaw's error

mye1 = mcy - mry;
if mye1 <= 0
    mye2 = mye1 + 360;
else
    mye2 = mye1 - 360;
end

if abs(mye1) <= abs(mye2);
    mye = mye1;
else
    mye = mye2;
end

== matlab function MAIN_UAVSIM_Simulink/controller/Waypoint Controller/Detect Roll Limiter Status ==
  data: wr_stat input; wr_stat output; cur_roll input
function wr_stat = fcn(wr_stat, cur_roll)
    if cur_roll >=30
        wr_stat = 1;
    end
end

== matlab function MAIN_UAVSIM_Simulink/controller/Waypoint Controller/PID & Model ANN/Controller Data Selection PID ==
  data: cur_roll input; r_lim input; y output; y_pid input; errYaw input; wl input
function y = fcn(cur_roll,r_lim,y_pid,errYaw,wl)
%#eml
%diff

if abs(cur_roll)>=30
    y = r_lim;
else
    y = double(y_pid);
end
end

== matlab function MAIN_UAVSIM_Simulink/controller/Waypoint Controller/heading angle modifier ==
  data: cur_yaw input; mcy output
function mcy = fcn(cur_yaw)
%#eml
% mcy = modified current yaw
mcy = cur_yaw;

if cur_yaw >= 180
    mcy = cur_yaw - 360;
end

== matlab function MAIN_UAVSIM_Simulink/controller/Waypoint Controller/heading angle modifier1 ==
  data: ref_yaw input; myr output
function myr = fcn(ref_yaw)
%#eml
% myr = modified ref. yaw

myr = ref_yaw;

if ref_yaw >= 180
    myr = ref_yaw - 360;  
end
